simulink model "bayesian_th"  (R2018b)
settings: Solver=ode45  StartTime=0.0  StopTime=simTimeBa  FixedStep=0.05  MaxStep=maxStep  RelTol=1e-3
values from neighbouring files (symbols this model uses):
  Cp = 0.6    [bayesian_ts.m]
  downstreamTurbPos = td*[7;0;0]    [bayesian_ts.m]    (also in wakeDeflection_ts.m)
  dt = 20    [bayesian_ts.m]
  rhoF = 1    [bayesian_ts.m]
  td = 0.15    [bayesian_ts.m]    (also in wakeDeflection_ts.m)
  upstreamTurbFlow = 4    [bayesian_ts.m]    (also in wakeDeflection_ts.m)
  upstreamTurbPos = [0;0;0]    [bayesian_ts.m]    (also in wakeDeflection_ts.m)
libraries: windTurbine_ul x1, bayesianAscent2_cl x1, wakeDeflection_ul x1
settings Model: Creator=asiddiq2  LastModifiedBy=Ayaz

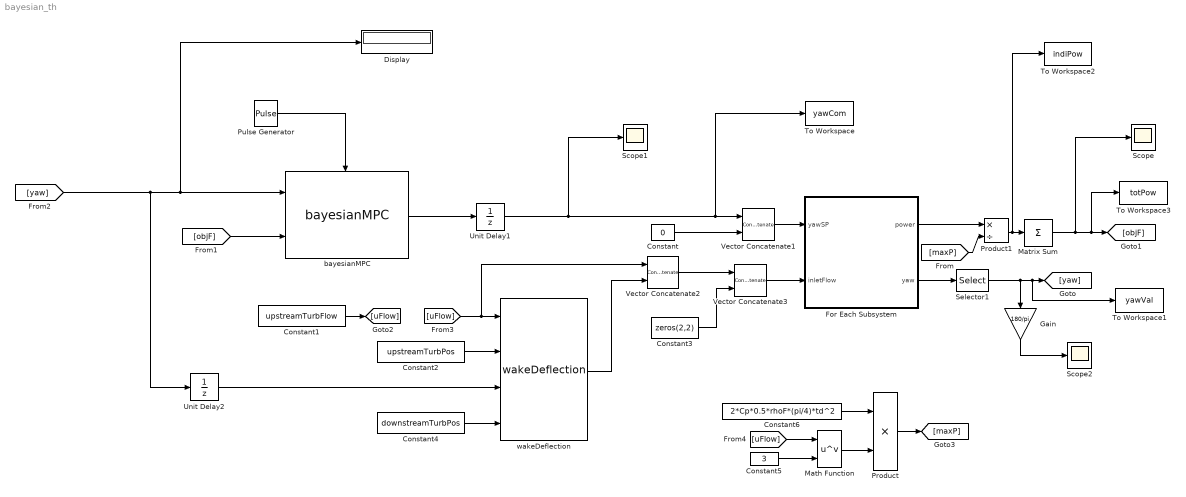
== system bayesian_th ==
  Constant : Constant  Value=0
  Constant1 : Constant  Value=upstreamTurbFlow  VectorParams1D=off
  Constant2 : Constant  Value=upstreamTurbPos  VectorParams1D=off
  Constant3 : Constant  Value=zeros(2,2)  VectorParams1D=off
  Constant4 : Constant  Value=downstreamTurbPos  VectorParams1D=off
  Constant5 : Constant  Value=3
  Constant6 : Constant  Value=2*Cp*0.5*rhoF*(pi/4)*td^2
  Display : Display
  For Each Subsystem : Subsystem  TreatAsAtomicUnit=on
  Gain : Gain  Gain=180/pi
  Math Function : Math  Operator=pow  SaturateOnIntegerOverflow=on
  Matrix Sum : Sum  Inputs=+
  Product : Product
  Product1 : Product  Inputs=*/
  Pulse Generator : DiscretePulseGenerator  PulseType=Time based  Period=dt  PulseWidth=5
  Scope : Scope
  Scope1 : Scope
  Scope2 : Scope
  Selector1 : Selector  InputPortWidth=2  IndexOptions=Index vector (dialog)  Indices=1  OutputSizes=1
  To Workspace : ToWorkspace  VariableName=yawCom  SaveFormat=Timeseries  SampleTime=-1
  To Workspace1 : ToWorkspace  VariableName=yawVal  SaveFormat=Timeseries  SampleTime=-1
  To Workspace2 : ToWorkspace  VariableName=indiPow  SaveFormat=Timeseries  SampleTime=-1
  To Workspace3 : ToWorkspace  VariableName=totPow  SaveFormat=Timeseries  SampleTime=-1
  Unit Delay1 : UnitDelay  SampleTime=-1
  Unit Delay2 : UnitDelay  SampleTime=-1
  Vector Concatenate1 : Concatenate  Mode=Multidimensional array  ConcatenateDimension=2
  Vector Concatenate2 : Concatenate  Mode=Multidimensional array  ConcatenateDimension=2
  Vector Concatenate3 : Concatenate  Mode=Multidimensional array
  bayesianMPC : bayesianAscent2_cl/bayesianMPC  gpModel=gp  gpTrain=trainDsgn  gpTrainFval=trainFval  desLims=designLimits  gamma=0.01  beta=1.1  iniTauPerc=0.25  maxIter=maxIter  predHorz=3  ctrlHorz=1
  wakeDeflection : wakeDeflection_ul/wakeDeflection  nTheta=nd  nD=nth  turbDia=td  ky=ky  kz=kz  CT=CT
  wires:
  Selector1/1 -> Gain/1, To Workspace1/1, [yaw]
  Vector Concatenate2/1 -> Vector Concatenate3/1
  Constant3/1 -> Vector Concatenate3/2
  [uFlow] -> Vector Concatenate2/1, wakeDeflection/1
  Constant2/1 -> wakeDeflection/2
  Constant4/1 -> wakeDeflection/4
  wakeDeflection/1 -> Vector Concatenate2/2
  For Each Subsystem/2(yaw) -> Selector1/1
  Constant/1 -> Vector Concatenate1/2
  Vector Concatenate1/1 -> For Each Subsystem/1(yawSP)
  Vector Concatenate3/1 -> For Each Subsystem/2(inletFlow)
  [objF] -> bayesianMPC/2
  Pulse Generator/1 -> bayesianMPC/Trigger
  bayesianMPC/1 -> Unit Delay1/1
  Gain/1 -> Scope2/1
  Constant1/1 -> [uFlow]
  Product/1 -> [maxP]
  Constant6/1 -> Product/1
  Math Function/1 -> Product/2
  [uFlow] -> Math Function/1
  Constant5/1 -> Math Function/2
  Matrix Sum/1 -> Scope/1, To Workspace3/1, [objF]
  [yaw] -> Unit Delay2/1, bayesianMPC/1, Display/1
  Unit Delay1/1 -> Scope1/1, To Workspace/1, Vector Concatenate1/1
  Unit Delay2/1 -> wakeDeflection/3
  Product1/1 -> To Workspace2/1, Matrix Sum/1
  [maxP] -> Product1/2
  For Each Subsystem/1(power) -> Product1/1

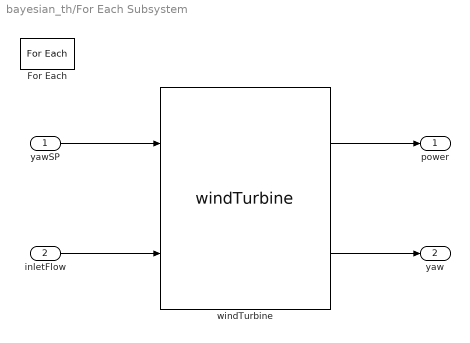
== system bayesian_th/For Each Subsystem ==
  yawSP : Inport  Partition=on  PartitionDimension=2  PartitionWidth=1  PartitionOffset=0
  inletFlow : Inport  Port=2  Partition=on  PartitionDimension=2  PartitionWidth=1  PartitionOffset=0
  For Each : ForEach  DisableCoverage=on  IndexMode=One-based
  windTurbine : windTurbine_ul/windTurbine  Cp=Cp  rhoFluid=rhoF  diam=td  Izz=Izz  iniYaw=0  gainMat="[95.0000   55.0000   50.0000]"
  power : Outport  ConcatenationDimension=2
  yaw : Outport  Port=2  ConcatenationDimension=2
  wires:
  yawSP/1 -> windTurbine/1
  inletFlow/1 -> windTurbine/2
  windTurbine/1 -> power/1
  windTurbine/2 -> yaw/1
